simulink model "TinBotIntroducer"  (Simulink 8.7)
settings: Solver=VariableStepAuto  StartTime=0.0  StopTime=1.8  MaxStep=0.001  RelTol=1e-3
libraries: simulink x2
settings Model: Creator=maximilian  LastModifiedBy=maximilian
settings DataIOCC: LimitDataPoints=off  SaveFormat=Dataset
settings DebuggingCC: UnderspecifiedInitializationDetection=Simplified  MergeDetectMultiDrivingBlocksExec=error
settings HardwareCC: ProdBitPerPointer=64  ProdLargestAtomicFloat=Float  ProdIntDivRoundTo=Zero  ProdEndianess=LittleEndian  ProdWordSize=64  ProdHWDeviceType=Intel->x86-64 (Windows64)
settings ModelReferenceCC: PropagateSignalLabelsOutOfModel=on
settings ConfigComp: CovModelRefEnable=off

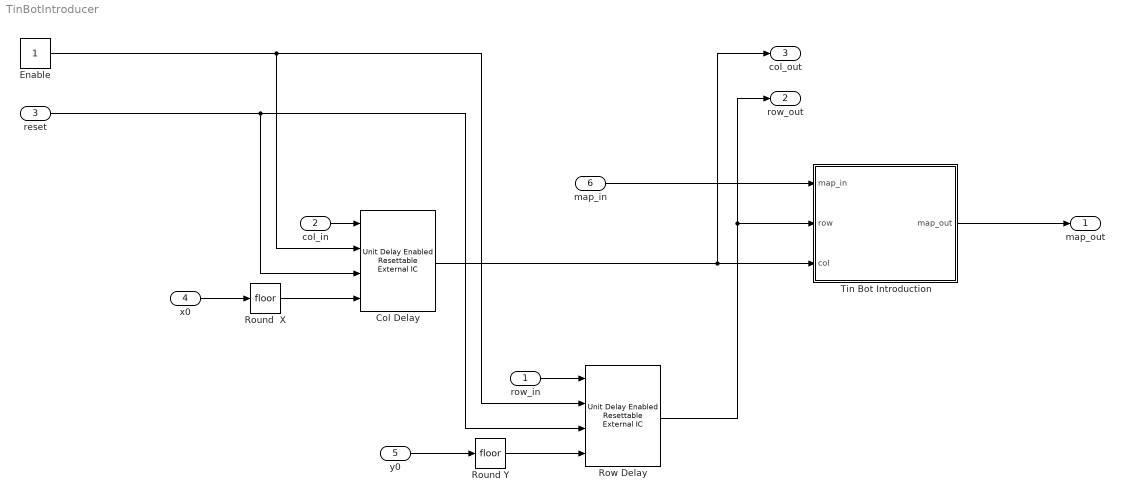
== system TinBotIntroducer ==
  row_in : Inport  Interpolate=off
  col_in : Inport  Port=2  Interpolate=off
  reset : Inport  Port=3
  x0 : Inport  Port=4
  y0 : Inport  Port=5
  map_in : Inport  Port=6  PortDimensions=[100 100]  Interpolate=off
  Col Delay : simulink/Additional Math & Discrete/Additional Discrete/Unit Delay Enabled Resettable External IC  tsamp=0.001
  Enable : Constant
  Round  X : Rounding
  Round Y : Rounding
  Row Delay : simulink/Additional Math & Discrete/Additional Discrete/Unit Delay Enabled Resettable External IC  tsamp=0.001
  Tin Bot Introduction : MATLAB Function  TreatAsAtomicUnit=on
  map_out : Outport  PortDimensions=[100 100]
  row_out : Outport  Port=2
  col_out : Outport  Port=3
  wires:
  reset/1 -> Row Delay/3, Col Delay/3
  y0/1 -> Round Y/1
  Round Y/1 -> Row Delay/4
  Round  X/1 -> Col Delay/4
  x0/1 -> Round  X/1
  Enable/1 -> Row Delay/2, Col Delay/2
  col_in/1 -> Col Delay/1
  row_in/1 -> Row Delay/1
  Col Delay/1 -> col_out/1, Tin Bot Introduction/3(col)
  Row Delay/1 -> row_out/1, Tin Bot Introduction/2(row)
  map_in/1 -> Tin Bot Introduction/1(map_in)
  Tin Bot Introduction/1(map_out) -> map_out/1

== matlab function Tin Bot Introduction ==
  data: map_in input double; map_out output double; row input double; col input double
function map_out = introduce(map_in, row, col)
    map_in(row, col) = 3;
    map_out = map_in;
